simulink model "modelo_completo"  (R2015b)
settings: Solver=ode4  StartTime=0.0  StopTime=t_sim  FixedStep=.001  RelTol=1e-3
values from neighbouring files (symbols this model uses):
  a1 = 0.0135    [modelo_completo_bueno3.m]
  a2 = 0.02    [modelo_completo_bueno3.m]
  A_e = double(eval(A))    [modelo_completo_bueno3.m]
  b1 = 0.0924    [modelo_completo_bueno3.m]
  B1phi = 1e-1    (= 0.1)    [modelo_completo_bueno3.m]
  B1psi = 6e-3    (= 0.006)    [modelo_completo_bueno3.m]
  b2 = 0.09    [modelo_completo_bueno3.m]
  B2phi = 1e-2    (= 0.01)    [modelo_completo_bueno3.m]
  B2psi = 1e-3    (= 0.001)    [modelo_completo_bueno3.m]
  B_e = double(eval(B))    [modelo_completo_bueno3.m]
  C_e = double(eval(C))    [modelo_completo_bueno3.m]
  cond_ini = double([ x1 x2 x3 x4 x5 x6 x7]')    [modelo_completo_bueno3.m]    (also in sim_modelo_completo.m)
  D_e = double(eval(D))    [modelo_completo_bueno3.m]
  I1 = 6.8e-2    (= 0.068)    [modelo_completo_bueno3.m]
  I2 = 2e-2    (= 0.02)    [modelo_completo_bueno3.m]
  incremento_u_11 = 0.1    [modelo_completo_bueno3.m]    (also in sim_modelo_completo.m)
  incremento_u_22 = 0.1    [modelo_completo_bueno3.m]    (also in sim_modelo_completo.m)
  k1 = 1.1    [modelo_completo_bueno3.m]
  k2 = 0.8    [modelo_completo_bueno3.m]
  kc = -0.2    [modelo_completo_bueno3.m]
  Kgy = 0.05    [modelo_completo_bueno3.m]
  Mg = 0.32    [modelo_completo_bueno3.m]
  T0 = 3.5    [modelo_completo_bueno3.m]
  T10 = 1    [modelo_completo_bueno3.m]
  T11 = 1.1    [modelo_completo_bueno3.m]
  T20 = 1    [modelo_completo_bueno3.m]
  T21 = 1    [modelo_completo_bueno3.m]
  Tp = 2    [modelo_completo_bueno3.m]
  u_11 = double(u1_ini)    [modelo_completo_bueno3.m]    (also in sim_modelo_completo.m)
  u_22 = double(u2_ini)    [modelo_completo_bueno3.m]    (also in sim_modelo_completo.m)
settings Model: Creator=kaiser  LastModifiedBy=kaiser
settings DebuggingCC: MaxConsecutiveZCsMsg=none

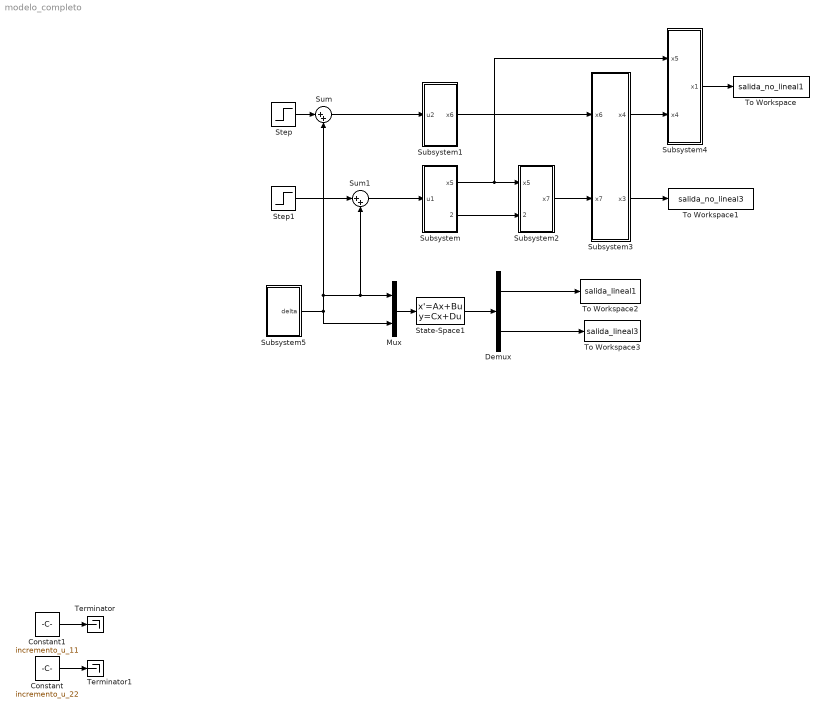
== system modelo_completo ==
  Constant : Constant  Value=incremento_u_22
  Constant1 : Constant  Value=incremento_u_11
  Demux : Demux  Outputs=2
  Mux : Mux  Inputs=2
  State-Space1 : StateSpace  A=A_e  B=B_e  C=C_e  D=D_e  X0=0
  Step : Step  Time=0  After=u_22  SampleTime=0
  Step1 : Step  Time=0  After=u_11  SampleTime=0
  Subsystem : Subsystem
  Subsystem1 : Subsystem
  Subsystem2 : Subsystem
  Subsystem3 : Subsystem
  Subsystem4 : Subsystem
  Subsystem5 : Subsystem
  Sum : Sum  Inputs=|++
  Sum1 : Sum  Inputs=|++
  Terminator : Terminator
  Terminator1 : Terminator
  To Workspace : ToWorkspace  VariableName=salida_no_lineal1  SaveFormat=Timeseries  SampleTime=-1
  To Workspace1 : ToWorkspace  VariableName=salida_no_lineal3  SaveFormat=Timeseries  SampleTime=-1
  To Workspace2 : ToWorkspace  VariableName=salida_lineal1  SaveFormat=Timeseries  SampleTime=-1
  To Workspace3 : ToWorkspace  VariableName=salida_lineal3  SaveFormat=Timeseries  SampleTime=-1
  wires:
  Subsystem/1(x5) -> Subsystem4/1(x5), Subsystem2/1(x5)
  Subsystem/2(x5_p) -> Subsystem2/2(x5_p)
  Subsystem1/1(x6) -> Subsystem3/1(x6)
  Subsystem2/1(x7) -> Subsystem3/2(x7)
  Subsystem3/1(x4) -> Subsystem4/2(x4)
  Subsystem4/1(x1) -> To Workspace/1
  Subsystem3/2(x3) -> To Workspace1/1
  Step/1 -> Sum/1
  Sum/1 -> Subsystem1/1(u2)
  Step1/1 -> Sum1/1
  Mux/1 -> State-Space1/1
  Demux/1 -> To Workspace2/1
  Demux/2 -> To Workspace3/1
  State-Space1/1 -> Demux/1
  Sum1/1 -> Subsystem/1(u1)
  Subsystem5/1(delta) -> Sum/2, Mux/1, Sum1/2, Mux/2
  Constant1/1 -> Terminator/1
  Constant/1 -> Terminator1/1

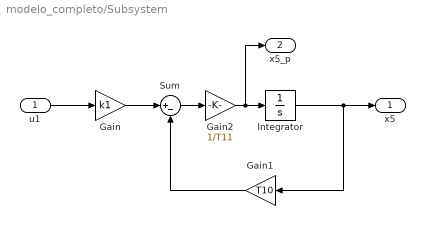
== system modelo_completo/Subsystem ==
  u1 : Inport
  Gain : Gain  Gain=k1
  Gain1 : Gain  Gain=T10
  Gain2 : Gain  Gain=1/T11
  Integrator : Integrator  InitialCondition=cond_ini(5)
  Sum : Sum  Inputs=|+-
  x5 : Outport
  x5_p : Outport  Port=2
  wires:
  Gain/1 -> Sum/1
  u1/1 -> Gain/1
  Integrator/1 -> x5/1, Gain1/1
  Gain1/1 -> Sum/2
  Sum/1 -> Gain2/1
  Gain2/1 -> x5_p/1, Integrator/1

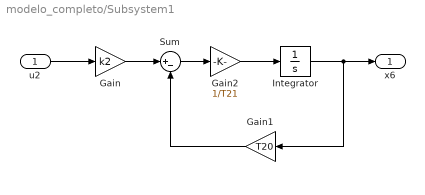
== system modelo_completo/Subsystem1 ==
  u2 : Inport
  Gain : Gain  Gain=k2
  Gain1 : Gain  Gain=T20
  Gain2 : Gain  Gain=1/T21
  Integrator : Integrator  InitialCondition=cond_ini(6)
  Sum : Sum  Inputs=|+-
  x6 : Outport
  wires:
  Gain2/1 -> Integrator/1
  Sum/1 -> Gain2/1
  Gain1/1 -> Sum/2
  Integrator/1 -> Gain1/1, x6/1
  u2/1 -> Gain/1
  Gain/1 -> Sum/1

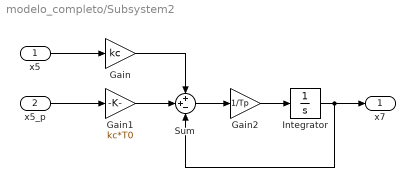
== system modelo_completo/Subsystem2 ==
  x5 : Inport
  x5_p : Inport  Port=2
  Gain : Gain  Gain=kc
  Gain1 : Gain  Gain=kc*T0
  Gain2 : Gain  Gain=1/Tp
  Integrator : Integrator  InitialCondition=cond_ini(7)
  Sum : Sum  Inputs=++-
  x7 : Outport
  wires:
  x5/1 -> Gain/1
  x5_p/1 -> Gain1/1
  Gain1/1 -> Sum/2
  Gain/1 -> Sum/1
  Integrator/1 -> Sum/3, x7/1
  Sum/1 -> Gain2/1
  Gain2/1 -> Integrator/1

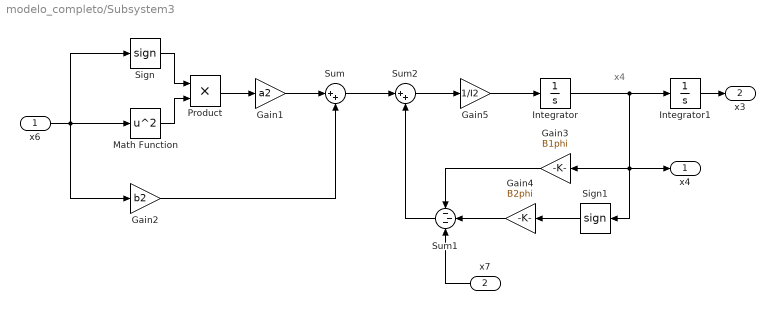
== system modelo_completo/Subsystem3 ==
  note: x4
  x6 : Inport
  x7 : Inport  Port=2
  Gain1 : Gain  Gain=a2
  Gain2 : Gain  Gain=b2
  Gain3 : Gain  Gain=B1phi
  Gain4 : Gain  Gain=B2phi
  Gain5 : Gain  Gain=1/I2
  Integrator : Integrator  InitialCondition=cond_ini(4)
  Integrator1 : Integrator  InitialCondition=cond_ini(3)
  Math Function : Math  Operator=square  OutputSignalType=real  SaturateOnIntegerOverflow=on
  Product : Product
  Sign : Signum  ZeroCross=off
  Sign1 : Signum  ZeroCross=off
  Sum : Sum  Inputs=|++
  Sum1 : Sum  Inputs=---
  Sum2 : Sum  Inputs=|++
  x4 : Outport
  x3 : Outport  Port=2
  wires:
  x6/1 -> Gain2/1, Sign/1, Math Function/1
  Sign/1 -> Product/1
  Math Function/1 -> Product/2
  Product/1 -> Gain1/1
  Gain2/1 -> Sum/2
  Gain1/1 -> Sum/1
  Integrator/1 -> Integrator1/1, x4/1, Sign1/1, Gain3/1
  Sign1/1 -> Gain4/1
  x7/1 -> Sum1/3
  Gain4/1 -> Sum1/2
  Gain3/1 -> Sum1/1
  Sum/1 -> Sum2/1
  Sum1/1 -> Sum2/2
  Sum2/1 -> Gain5/1
  Gain5/1 -> Integrator/1
  Integrator1/1 -> x3/1

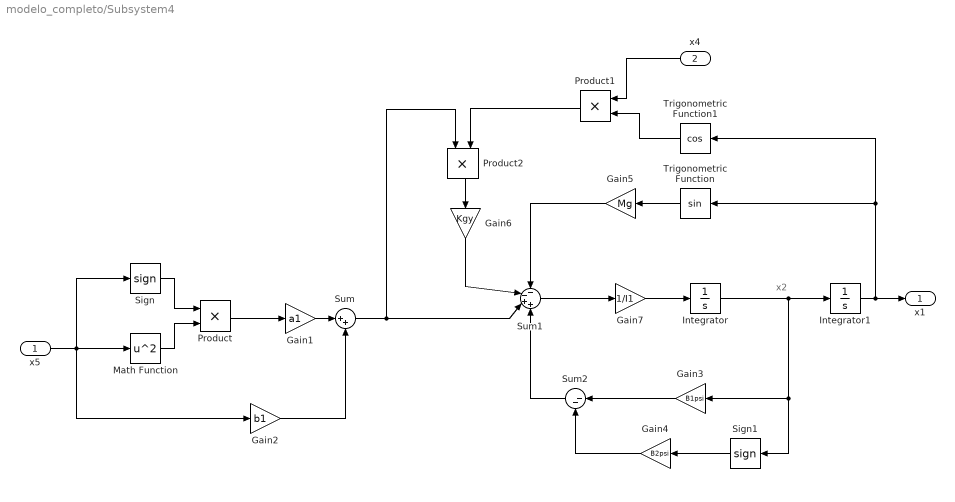
== system modelo_completo/Subsystem4 ==
  note: x2
  x5 : Inport
  x4 : Inport  Port=2
  Gain1 : Gain  Gain=a1
  Gain2 : Gain  Gain=b1
  Gain3 : Gain  Gain=B1psi
  Gain4 : Gain  Gain=B2psi
  Gain5 : Gain  Gain=Mg
  Gain6 : Gain  Gain=Kgy
  Gain7 : Gain  Gain=1/I1
  Integrator : Integrator  InitialCondition=cond_ini(2)
  Integrator1 : Integrator  InitialCondition=cond_ini(1)
  Math Function : Math  Operator=square  OutputSignalType=real  SaturateOnIntegerOverflow=on
  Product : Product
  Product1 : Product
  Product2 : Product
  Sign : Signum  ZeroCross=off
  Sign1 : Signum  ZeroCross=off
  Sum : Sum  Inputs=|++
  Sum1 : Sum  Inputs=--++
  Sum2 : Sum  Inputs=|--
  Trigonometric Function : Trigonometry
  Trigonometric Function1 : Trigonometry  Operator=cos
  x1 : Outport
  wires:
  x5/1 -> Gain2/1, Sign/1, Math Function/1
  Sign/1 -> Product/1
  Math Function/1 -> Product/2
  Product/1 -> Gain1/1
  Gain2/1 -> Sum/2
  Gain1/1 -> Sum/1
  Sign1/1 -> Gain4/1
  Integrator/1 -> Integrator1/1, Sign1/1, Gain3/1
  Integrator1/1 -> Trigonometric Function/1, Trigonometric Function1/1, x1/1
  Trigonometric Function/1 -> Gain5/1
  Sum/1 -> Product2/1, Sum1/3
  Gain5/1 -> Sum1/1
  Gain4/1 -> Sum2/2
  Gain3/1 -> Sum2/1
  Trigonometric Function1/1 -> Product1/2
  x4/1 -> Product1/1
  Product1/1 -> Product2/2
  Product2/1 -> Gain6/1
  Gain6/1 -> Sum1/2
  Sum2/1 -> Sum1/4
  Sum1/1 -> Gain7/1
  Gain7/1 -> Integrator/1

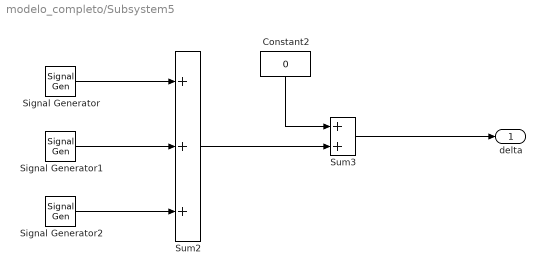
== system modelo_completo/Subsystem5 ==
  Constant2 : Constant  Value=0
  Signal Generator : SignalGenerator  Amplitude=0.1  Frequency=0.1
  Signal Generator1 : SignalGenerator  Amplitude=0.1  Frequency=0.05
  Signal Generator2 : SignalGenerator  Amplitude=0.1  Frequency=0.02
  Sum2 : Sum  Inputs=+++
  Sum3 : Sum
  delta : Outport
  wires:
  Sum2/1 -> Sum3/2
  Signal Generator1/1 -> Sum2/2
  Signal Generator2/1 -> Sum2/3
  Constant2/1 -> Sum3/1
  Sum3/1 -> delta/1
  Signal Generator/1 -> Sum2/1
